simulink model "generatoreqns"  (Simulink 7.6)
settings: Solver=ode45  StartTime=0.0  StopTime=50  RelTol=1e-3
settings Model: Creator=Renata  LastModifiedBy=Renata

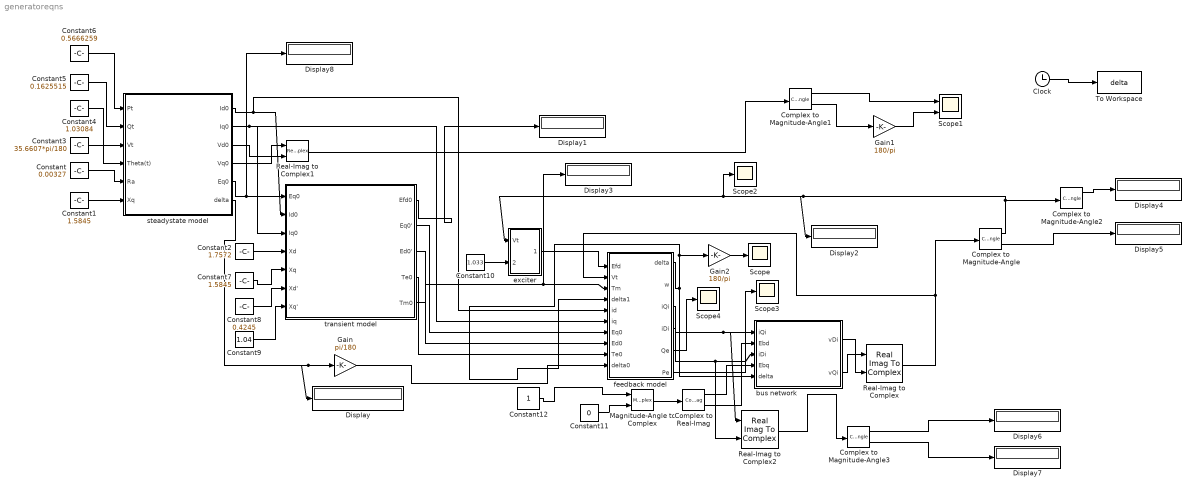
== system generatoreqns ==
  Clock : Clock
      settings: Decimation=10
  Complex to Magnitude-Angle{,1..3} (4 alike) : ComplexToMagnitudeAngle
  Complex to Real-Imag : ComplexToRealImag
  Constant : Constant  Value=0.00327
  Constant1 : Constant  Value=1.5845
  Constant10 : Constant  Value=1.033
  Constant11 : Constant  Value=0
  Constant12 : Constant
  Constant2 : Constant  Value=1.7572
  Constant3 : Constant  Value=35.6607*pi/180
  Constant4 : Constant  Value=1.03084
  Constant5 : Constant  Value=0.1625515
  Constant6 : Constant  Value=0.5666259
  Constant7 : Constant  Value=1.5845
  Constant8 : Constant  Value=0.4245
  Constant9 : Constant  Value=1.04
  Display{,1..8} (9 alike) : Display
  Gain : Gain  Gain=pi/180
  Gain1 : Gain  Gain=180/pi
  Gain2 : Gain  Gain=180/pi
  Magnitude-Angle to Complex : MagnitudeAngleToComplex
  Real-Imag to Complex : RealImagToComplex
  Real-Imag to Complex1 : RealImagToComplex
  Real-Imag to Complex2 : RealImagToComplex
  Scope{,2..4} (4 alike) : Scope
      Scope settings: TickLabels=on  TimeRange=50  YMin=0.85  YMax=1.35
      Scope2 settings: TickLabels=on  TimeRange=50  YMin=0.85  YMax=1.35  SaveName=ScopeData2
      Scope3 settings: TickLabels=on  TimeRange=50  YMin=0.85  YMax=1.35  SaveName=ScopeData3
      Scope4 settings: TickLabels=on  TimeRange=50  YMin=0.85  YMax=1.35  SaveName=ScopeData5
  Scope1 : Scope  NumInputPorts=2
      settings: YMin=-5~-5  YMax=5~5
  To Workspace : ToWorkspace  VariableName=delta  SampleTime=-1  SaveFormat=Structure
      settings: Decimation=100
  bus network : Subsystem
  exciter : Subsystem
  feedback model : Subsystem
  steadystate model : Subsystem
  transient model : Subsystem
  wires:
  steadystate model/1(Id0) -> transient model/2(Id0), feedback model/5(id)
  steadystate model/2(Iq0) -> transient model/3(Iq0), feedback model/6(iq)
  steadystate model/5(Eq0) -> transient model/1(Eq0), Display8/1
  Constant/1 -> steadystate model/5(Ra)
  Constant1/1 -> steadystate model/6(Xq)
  Constant3/1 -> steadystate model/4(Theta(t))
  Constant4/1 -> steadystate model/3(Vt)
  Constant5/1 -> steadystate model/2(Qt)
  Constant6/1 -> steadystate model/1(Pt)
  Constant2/1 -> transient model/4(Xd)
  Constant7/1 -> transient model/5(Xq)
  Constant8/1 -> transient model/6(Xd')
  Constant9/1 -> transient model/7(Xq')
  feedback model/1(delta) -> bus network/5(delta), feedback model/4(delta1), Gain2/1
  Constant10/1 -> exciter/2(Vref)
  feedback model/4(iDi) -> bus network/3(iDi), Real-Imag to Complex2/2
  bus network/1(vDi) -> Real-Imag to Complex/2
  bus network/2(vQi) -> Real-Imag to Complex/1
  Magnitude-Angle to Complex/1 -> Complex to Real-Imag/1
  Constant12/1 -> Magnitude-Angle to Complex/1
  Constant11/1 -> Magnitude-Angle to Complex/2
  Complex to Magnitude-Angle/1 -> Complex to Magnitude-Angle2/1, Display2/1, exciter/1(Vt), Scope2/1
  transient model/1(Efd0) -> Display1/1
  steadystate model/4(Vq0) -> Real-Imag to Complex1/1
  steadystate model/3(Vd0) -> Real-Imag to Complex1/2
  transient model/2(Eq0') -> feedback model/7(Eq0)
  transient model/3(Ed0') -> feedback model/8(Ed0)
  transient model/4(Te0) -> feedback model/9(Te0)
  Real-Imag to Complex1/1 -> Complex to Magnitude-Angle1/1
  steadystate model/6(delta) -> Gain/1, Display/1
  Gain/1 -> feedback model/10(delta0)
  Complex to Magnitude-Angle1/1 -> Scope1/1
  Complex to Magnitude-Angle1/2 -> Gain1/1
  Gain1/1 -> Scope1/2
  feedback model/3(iQi) -> bus network/1(iQi), Real-Imag to Complex2/1
  Real-Imag to Complex/1 -> Complex to Magnitude-Angle/1, feedback model/2(Vt)
  transient model/5(Tm0) -> feedback model/3(Tm), Display3/1
  Complex to Real-Imag/2 -> bus network/2(Ebd)
  Complex to Real-Imag/1 -> bus network/4(Ebq)
  Complex to Magnitude-Angle2/1 -> Display4/1
  Complex to Magnitude-Angle/2 -> Display5/1
  Real-Imag to Complex2/1 -> Complex to Magnitude-Angle3/1
  Complex to Magnitude-Angle3/2 -> Display7/1
  Complex to Magnitude-Angle3/1 -> Display6/1
  Clock/1 -> To Workspace/1
  feedback model/6(Pe) -> Scope3/1
  feedback model/5(Qe) -> Scope4/1
  Gain2/1 -> Scope/1
  exciter/1(Efd) -> feedback model/1(Efd)

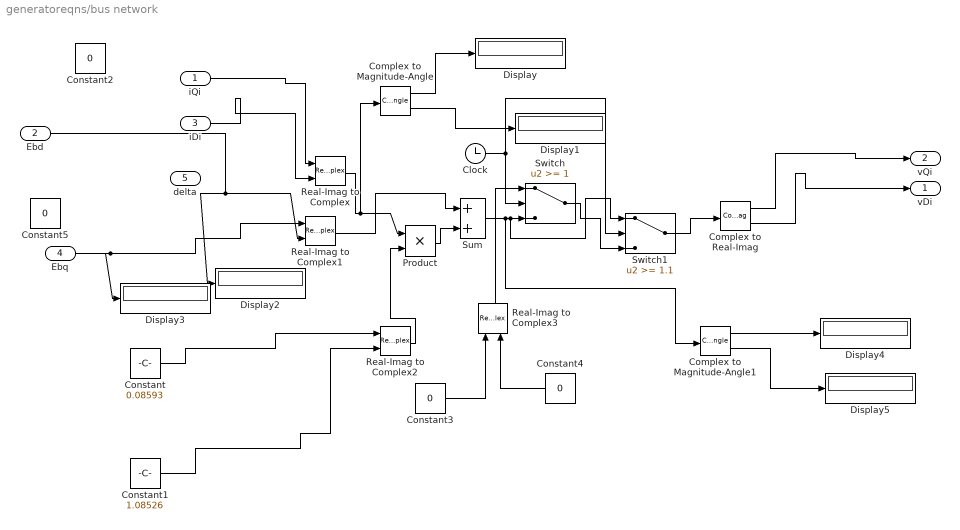
== system generatoreqns/bus network ==
  iQi : Inport
  Ebd : Inport  Port=2
  iDi : Inport  Port=3
  Ebq : Inport  Port=4
  delta : Inport  Port=5
  Clock : Clock
      settings: Decimation=1000
  Complex to Magnitude-Angle : ComplexToMagnitudeAngle
  Complex to Magnitude-Angle1 : ComplexToMagnitudeAngle
  Complex to Real-Imag : ComplexToRealImag
  Constant : Constant  Value=0.08593
  Constant1 : Constant  Value=1.08526
  Constant{2..5} (4 alike) : Constant  Value=0
  Display{,1..5} (6 alike) : Display
  Product : Product  RndMeth=Zero
  Real-Imag to Complex{,1..3} (4 alike) : RealImagToComplex
  Sum : Sum  Inputs=|++
  Switch : Switch  Threshold=1
  Switch1 : Switch  Threshold=1.1
  vDi : Outport
  vQi : Outport  Port=2
  wires:
  Real-Imag to Complex/1 -> Product/1, Complex to Magnitude-Angle/1
  Real-Imag to Complex2/1 -> Product/2
  Product/1 -> Sum/2
  Real-Imag to Complex1/1 -> Sum/1
  Constant/1 -> Real-Imag to Complex2/1
  Constant1/1 -> Real-Imag to Complex2/2
  Switch/1 -> Switch1/3
  iQi/1 -> Real-Imag to Complex/1
  iDi/1 -> Real-Imag to Complex/2
  Clock/1 -> Switch/2, Switch1/2
  Sum/1 -> Complex to Magnitude-Angle1/1, Switch/3, Switch1/1
  Real-Imag to Complex3/1 -> Switch/1
  Constant4/1 -> Real-Imag to Complex3/2
  Constant3/1 -> Real-Imag to Complex3/1
  Complex to Real-Imag/1 -> vQi/1
  Complex to Real-Imag/2 -> vDi/1
  Ebq/1 -> Real-Imag to Complex1/1, Display3/1
  Ebd/1 -> Real-Imag to Complex1/2, Display2/1
  Complex to Magnitude-Angle/1 -> Display/1
  Complex to Magnitude-Angle/2 -> Display1/1
  Complex to Magnitude-Angle1/1 -> Display4/1
  Complex to Magnitude-Angle1/2 -> Display5/1
  Switch1/1 -> Complex to Real-Imag/1

== system generatoreqns/exciter ==
  Vt : Inport
  Vref : Inport  Port=2
  Saturation1 : Saturate  UpperLimit=1.5  LowerLimit=-1.5
  Sum : Sum  Inputs=|+-
  Transfer Fcn : TransferFcn  Numerator=[400]  Denominator=[0.025 1]
  Efd : Outport
  wires:
  Transfer Fcn/1 -> Saturation1/1
  Sum/1 -> Transfer Fcn/1
  Vt/1 -> Sum/1
  Vref/1 -> Sum/2
  Saturation1/1 -> Efd/1

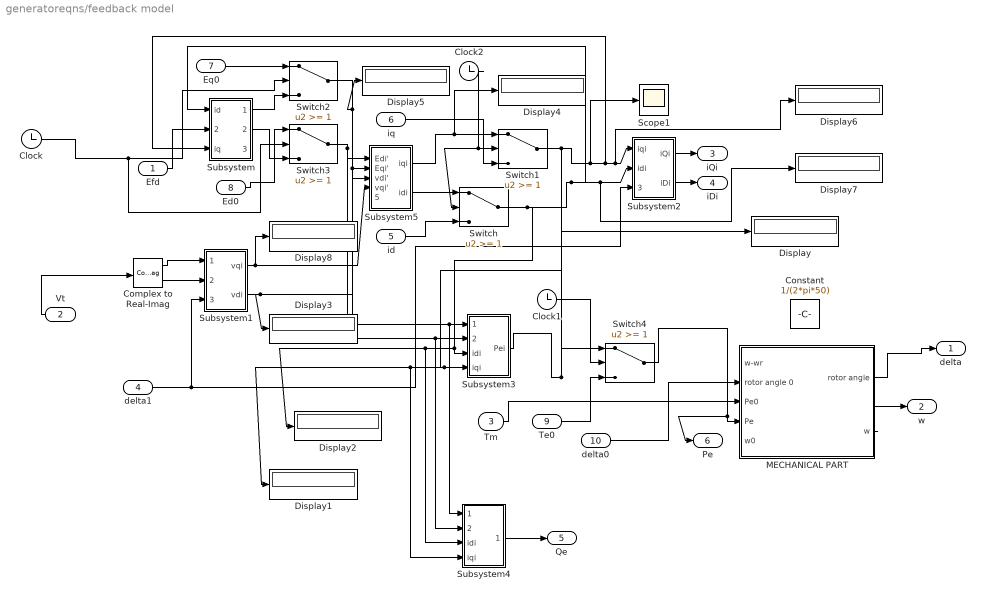
== system generatoreqns/feedback model ==
  Efd : Inport
  Vt : Inport  Port=2
  Tm : Inport  Port=3
  delta1 : Inport  Port=4
  id : Inport  Port=5
  iq : Inport  Port=6
  Eq0 : Inport  Port=7
  Ed0 : Inport  Port=8
  Te0 : Inport  Port=9
  delta0 : Inport  Port=10
  Clock : Clock
      settings: Decimation=1000
  Clock1 : Clock
      settings: Decimation=1000
  Clock2 : Clock
      settings: Decimation=1000
  Complex to Real-Imag : ComplexToRealImag
  Constant : Constant  Value=1/(2*pi*50)
  Display{,1..8} (9 alike) : Display
  MECHANICAL PART : Subsystem
  Scope1 : Scope
      settings: SaveName=ScopeData4
  Subsystem : Subsystem
  Subsystem1 : Subsystem
  Subsystem2 : Subsystem
  Subsystem3 : Subsystem
  Subsystem4 : Subsystem
  Subsystem5 : Subsystem
  Switch{,1..3} (4 alike) : Switch  Threshold=1
  Switch4 : Switch  Threshold=1  ZeroCross=off
  delta : Outport
  w : Outport  Port=2
  iQi : Outport  Port=3
  iDi : Outport  Port=4
  Qe : Outport  Port=5
  Pe : Outport  Port=6
  wires:
  Complex to Real-Imag/1 -> Subsystem1/1(VQi)
  Complex to Real-Imag/2 -> Subsystem1/2(VDi)
  Efd/1 -> Subsystem/2(Efd)
  Vt/1 -> Complex to Real-Imag/1
  Tm/1 -> MECHANICAL PART/3(Pe0)
  Subsystem2/1(iQi) -> iQi/1
  Subsystem2/2(iDi) -> iDi/1
  iq/1 -> Switch1/3
  Clock/1 -> Switch2/2, Switch3/2
  MECHANICAL PART/1(rotor angle) -> delta/1
  MECHANICAL PART/2(w) -> w/1
  delta0/1 -> MECHANICAL PART/2(rotor angle 0)
  Eq0/1 -> Switch2/1
  Subsystem/1(Eqi') -> Switch2/3
  Ed0/1 -> Switch3/1
  Subsystem/2(Edi') -> Switch3/3
  Subsystem5/2(idi) -> Switch/1
  id/1 -> Switch/3
  Subsystem5/1(iqi) -> Switch1/1, Display4/1
  Subsystem3/1(Pei) -> Display/1, Switch4/1
  Switch3/1 -> Subsystem5/1(Edi'), Subsystem3/1(Edi'), Subsystem4/1(Edi')
  Switch2/1 -> Subsystem5/2(Eqi'), Subsystem3/2(Eqi'), Subsystem4/2(Eqi'), Display5/1
  Subsystem1/1(vqi) -> Subsystem5/4(vqi'), Display8/1
  Subsystem1/2(vdi) -> Subsystem5/3(vdi'), Display3/1
  Switch/1 -> Subsystem/1(id), Subsystem2/2(idi), Display7/1, Subsystem3/3(idi), Display2/1, Subsystem4/3(idi)
  Switch1/1 -> Subsystem3/4(iqi), Display1/1, Subsystem4/4(iqi), Subsystem/3(iq), Subsystem2/1(iqi), Display6/1, Scope1/1
  Clock2/1 -> Switch1/2, Switch/2
  delta1/1 -> Subsystem1/3(delta), Subsystem2/3(delta)
  Subsystem4/1(Qei) -> Qe/1
  Te0/1 -> Switch4/3
  Clock1/1 -> Switch4/2
  Switch4/1 -> MECHANICAL PART/4(Pe), Pe/1

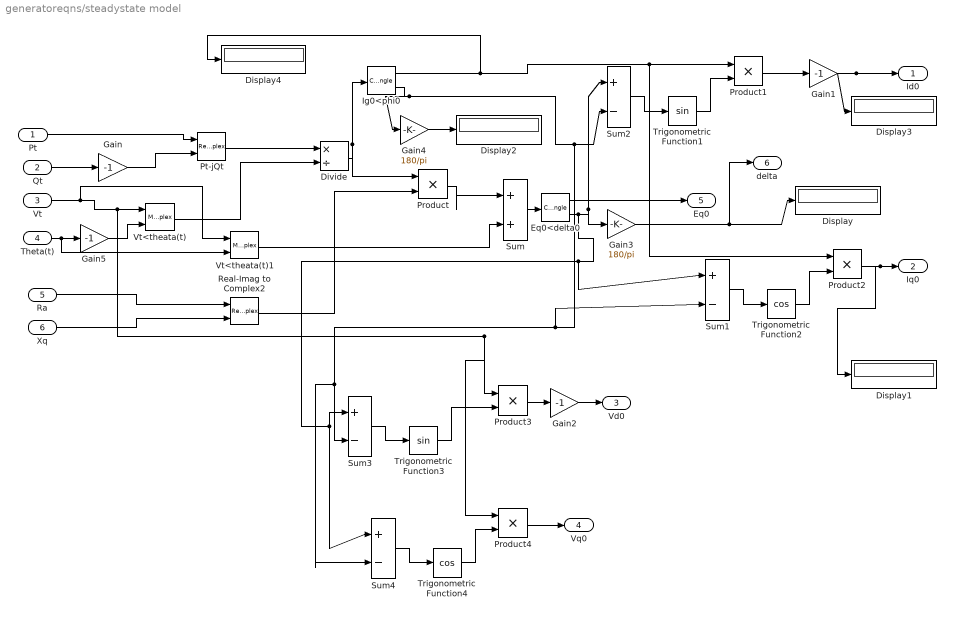
== system generatoreqns/steadystate model ==
  Pt : Inport
  Qt : Inport  Port=2
  Vt : Inport  Port=3
  Theta(t) : Inport  Port=4
  Ra : Inport  Port=5
  Xq : Inport  Port=6
  Display{,1..4} (5 alike) : Display
  Divide : Product  Inputs=*/  RndMeth=Round
  Eq0<delta0 : ComplexToMagnitudeAngle
  Gain{,1..2,5} (4 alike) : Gain  Gain=-1
  Gain3 : Gain  Gain=180/pi
  Gain4 : Gain  Gain=180/pi
  Ig0<phi0 : ComplexToMagnitudeAngle
  Product{,1..4} (5 alike) : Product  RndMeth=Zero
  Pt-jQt : RealImagToComplex
  Real-Imag to Complex2 : RealImagToComplex
  Sum : Sum  Inputs=|++
  Sum{1..4} (4 alike) : Sum  Inputs=|+-
  Trigonometric Function1 : Trigonometry
  Trigonometric Function2 : Trigonometry  Operator=cos
  Trigonometric Function3 : Trigonometry
  Trigonometric Function4 : Trigonometry  Operator=cos
  Vt<theata(t) : MagnitudeAngleToComplex
  Vt<theata(t)1 : MagnitudeAngleToComplex
  Id0 : Outport
  Iq0 : Outport  Port=2
  Vd0 : Outport  Port=3
  Vq0 : Outport  Port=4
  Eq0 : Outport  Port=5
  delta : Outport  Port=6
  wires:
  Qt/1 -> Gain/1
  Gain/1 -> Pt-jQt/2
  Pt/1 -> Pt-jQt/1
  Vt/1 -> Vt<theata(t)/1, Product3/1, Product4/1, Vt<theata(t)1/1
  Pt-jQt/1 -> Divide/1
  Vt<theata(t)/1 -> Divide/2
  Ra/1 -> Real-Imag to Complex2/1
  Xq/1 -> Real-Imag to Complex2/2
  Divide/1 -> Ig0<phi0/1, Product/1
  Real-Imag to Complex2/1 -> Product/2
  Product/1 -> Sum/1
  Sum/1 -> Eq0<delta0/1
  Eq0<delta0/2 -> Sum3/1, Sum4/1, Sum1/1, Sum2/1, Gain3/1
  Sum2/1 -> Trigonometric Function1/1
  Trigonometric Function1/1 -> Product1/2
  Ig0<phi0/1 -> Product1/1, Product2/1, Display4/1
  Product1/1 -> Gain1/1
  Gain1/1 -> Id0/1, Display3/1
  Sum1/1 -> Trigonometric Function2/1
  Trigonometric Function2/1 -> Product2/2
  Product2/1 -> Iq0/1, Display1/1
  Sum3/1 -> Trigonometric Function3/1
  Trigonometric Function3/1 -> Product3/2
  Product3/1 -> Gain2/1
  Gain2/1 -> Vd0/1
  Sum4/1 -> Trigonometric Function4/1
  Trigonometric Function4/1 -> Product4/2
  Product4/1 -> Vq0/1
  Eq0<delta0/1 -> Eq0/1
  Gain3/1 -> Display/1, delta/1
  Ig0<phi0/2 -> Sum2/2, Sum3/2, Sum4/2, Sum1/2, Gain4/1
  Theta(t)/1 -> Gain5/1, Vt<theata(t)1/2
  Gain5/1 -> Vt<theata(t)/2
  Vt<theata(t)1/1 -> Sum/2
  Gain4/1 -> Display2/1

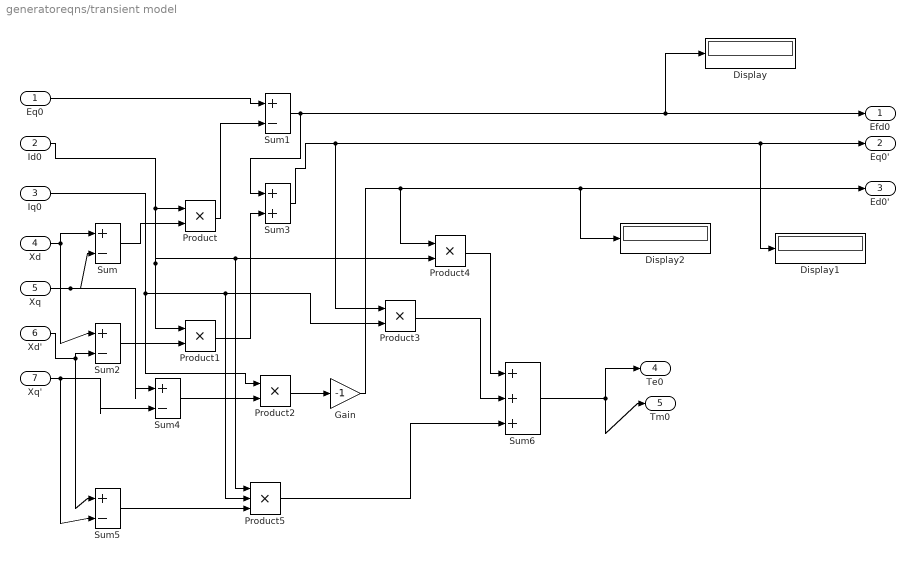
== system generatoreqns/transient model ==
  Eq0 : Inport
  Id0 : Inport  Port=2
  Iq0 : Inport  Port=3
  Xd : Inport  Port=4
  Xq : Inport  Port=5
  Xd' : Inport  Port=6
  Xq' : Inport  Port=7
  Display : Display
  Display1 : Display
  Display2 : Display
  Gain : Gain  Gain=-1
  Product{,1..4} (5 alike) : Product  RndMeth=Zero
  Product5 : Product  Inputs=3  RndMeth=Zero
  Sum{,1..2,4..5} (5 alike) : Sum  Inputs=|+-
  Sum3 : Sum  Inputs=|++
  Sum6 : Sum  Inputs=|+++
  Efd0 : Outport
  Eq0' : Outport  Port=2
  Ed0' : Outport  Port=3
  Te0 : Outport  Port=4
  Tm0 : Outport  Port=5
  wires:
  Sum6/1 -> Te0/1, Tm0/1
  Product5/1 -> Sum6/3
  Product3/1 -> Sum6/2
  Product4/1 -> Sum6/1
  Sum5/1 -> Product5/3
  Gain/1 -> Product4/1, Ed0'/1, Display2/1
  Product2/1 -> Gain/1
  Iq0/1 -> Product2/1, Product3/2, Product5/2
  Sum4/1 -> Product2/2
  Xq'/1 -> Sum4/2, Sum5/2
  Sum3/1 -> Product3/1, Eq0'/1, Display1/1
  Product1/1 -> Sum3/2
  Sum2/1 -> Product1/2
  Xd'/1 -> Sum2/2, Sum5/1
  Sum1/1 -> Sum3/1, Efd0/1, Display/1
  Product/1 -> Sum1/2
  Eq0/1 -> Sum1/1
  Id0/1 -> Product/1, Product1/1, Product4/2, Product5/1
  Sum/1 -> Product/2
  Xq/1 -> Sum/2, Sum4/1
  Xd/1 -> Sum/1, Sum2/1

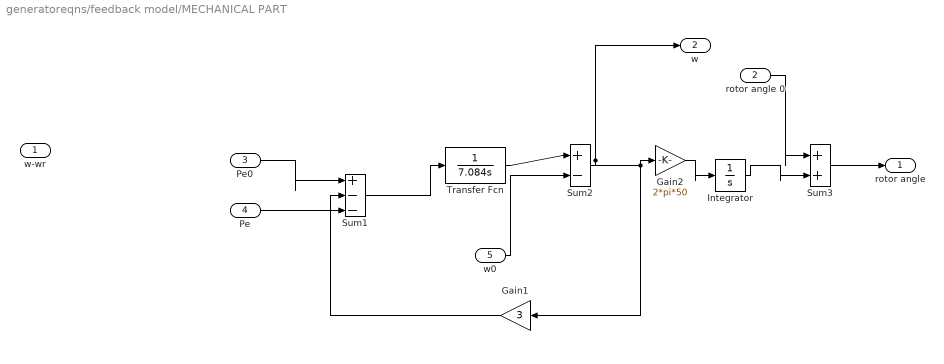
== system generatoreqns/feedback model/MECHANICAL PART ==
  w-wr : Inport
  rotor angle 0 : Inport  Port=2
  Pe0 : Inport  Port=3
  Pe : Inport  Port=4
  w0 : Inport  Port=5
  Gain1 : Gain  Gain=3
  Gain2 : Gain  Gain=2*pi*50
  Integrator : Integrator  ZeroCross=off
  Sum1 : Sum  Inputs=|+--
  Sum2 : Sum  Inputs=|+-
  Sum3 : Sum  Inputs=|++
  Transfer Fcn : TransferFcn  Denominator=[7.084 0]
  rotor angle : Outport
  w : Outport  Port=2
  wires:
  Sum1/1 -> Transfer Fcn/1
  Pe0/1 -> Sum1/1
  Pe/1 -> Sum1/2
  w0/1 -> Sum2/2
  Integrator/1 -> Sum3/2
  Sum3/1 -> rotor angle/1
  Sum2/1 -> w/1, Gain1/1, Gain2/1
  Transfer Fcn/1 -> Sum2/1
  Gain1/1 -> Sum1/3
  Gain2/1 -> Integrator/1
  rotor angle 0/1 -> Sum3/1

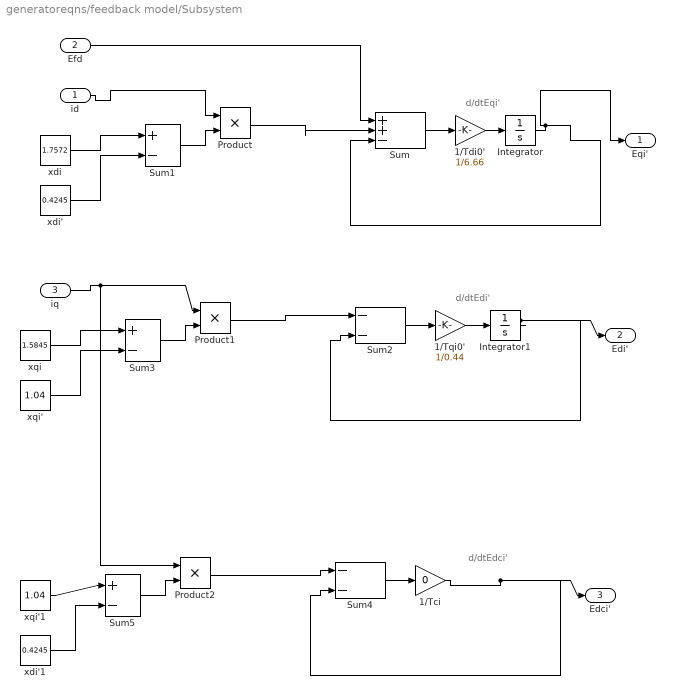
== system generatoreqns/feedback model/Subsystem ==
  note: d/dtEqi'
  note: d/dtEdi'
  note: d/dtEdci'
  id : Inport
  Efd : Inport  Port=2
  iq : Inport  Port=3
  1/Tci : Gain  Gain=0
  1/Tdi0' : Gain  Gain=1/6.66
  1/Tqi0' : Gain  Gain=1/0.44
  Integrator : Integrator
  Integrator1 : Integrator
  Product : Product  RndMeth=Zero
  Product1 : Product  RndMeth=Zero
  Product2 : Product  RndMeth=Zero
  Sum : Sum  Inputs=|++-
  Sum1 : Sum  Inputs=|+-
  Sum2 : Sum  Inputs=--
  Sum3 : Sum  Inputs=|+-
  Sum4 : Sum  Inputs=--
  Sum5 : Sum  Inputs=|+-
  xdi : Constant  Value=1.7572
  xdi' : Constant  Value=0.4245
  xdi'1 : Constant  Value=0.4245
  xqi : Constant  Value=1.5845
  xqi' : Constant  Value=1.04
  xqi'1 : Constant  Value=1.04
  Eqi' : Outport
  Edi' : Outport  Port=2
  Edci' : Outport  Port=3
  wires:
  Integrator/1 -> Eqi'/1, Sum/3
  xdi/1 -> Sum1/1
  xdi'/1 -> Sum1/2
  Sum1/1 -> Product/2
  id/1 -> Product/1
  Product/1 -> Sum/2
  Efd/1 -> Sum/1
  Sum/1 -> 1/Tdi0'/1
  1/Tdi0'/1 -> Integrator/1
  Integrator1/1 -> Edi'/1, Sum2/2
  xqi/1 -> Sum3/1
  xqi'/1 -> Sum3/2
  Sum3/1 -> Product1/2
  iq/1 -> Product1/1, Product2/1
  Sum2/1 -> 1/Tqi0'/1
  1/Tqi0'/1 -> Integrator1/1
  Product1/1 -> Sum2/1
  Sum5/1 -> Product2/2
  Sum4/1 -> 1/Tci/1
  1/Tci/1 -> Edci'/1, Sum4/2
  Product2/1 -> Sum4/1
  xqi'1/1 -> Sum5/1
  xdi'1/1 -> Sum5/2

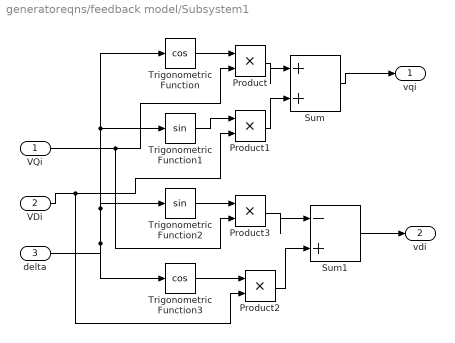
== system generatoreqns/feedback model/Subsystem1 ==
  VQi : Inport
  VDi : Inport  Port=2
  delta : Inport  Port=3
  Product{,1..3} (4 alike) : Product  RndMeth=Zero
  Sum : Sum  Inputs=|++
  Sum1 : Sum  Inputs=|-+
  Trigonometric Function : Trigonometry  Operator=cos
  Trigonometric Function1 : Trigonometry
  Trigonometric Function2 : Trigonometry
  Trigonometric Function3 : Trigonometry  Operator=cos
  vqi : Outport
  vdi : Outport  Port=2
  wires:
  Sum/1 -> vqi/1
  Sum1/1 -> vdi/1
  delta/1 -> Trigonometric Function/1, Trigonometric Function1/1, Trigonometric Function2/1, Trigonometric Function3/1
  Trigonometric Function/1 -> Product/1
  VQi/1 -> Product/2, Product3/2
  Product/1 -> Sum/1
  Trigonometric Function1/1 -> Product1/1
  VDi/1 -> Product1/2, Product2/2
  Product1/1 -> Sum/2
  Trigonometric Function2/1 -> Product3/1
  Trigonometric Function3/1 -> Product2/1
  Product3/1 -> Sum1/1
  Product2/1 -> Sum1/2

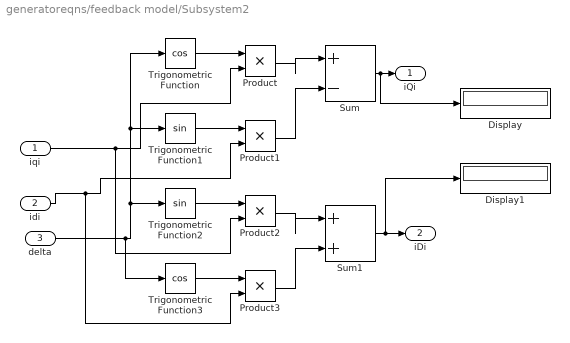
== system generatoreqns/feedback model/Subsystem2 ==
  iqi : Inport
  idi : Inport  Port=2
  delta : Inport  Port=3
  Display : Display
  Display1 : Display
  Product{,1..3} (4 alike) : Product  RndMeth=Zero
  Sum : Sum  Inputs=|+-
  Sum1 : Sum  Inputs=|++
  Trigonometric Function : Trigonometry  Operator=cos
  Trigonometric Function1 : Trigonometry
  Trigonometric Function2 : Trigonometry
  Trigonometric Function3 : Trigonometry  Operator=cos
  iQi : Outport
  iDi : Outport  Port=2
  wires:
  Sum1/1 -> iDi/1, Display1/1
  Sum/1 -> iQi/1, Display/1
  delta/1 -> Trigonometric Function/1, Trigonometric Function1/1, Trigonometric Function2/1, Trigonometric Function3/1
  Trigonometric Function/1 -> Product/1
  iqi/1 -> Product/2, Product2/2
  Product/1 -> Sum/1
  Trigonometric Function1/1 -> Product1/1
  idi/1 -> Product1/2, Product3/2
  Product1/1 -> Sum/2
  Trigonometric Function2/1 -> Product2/1
  Product2/1 -> Sum1/1
  Trigonometric Function3/1 -> Product3/1
  Product3/1 -> Sum1/2

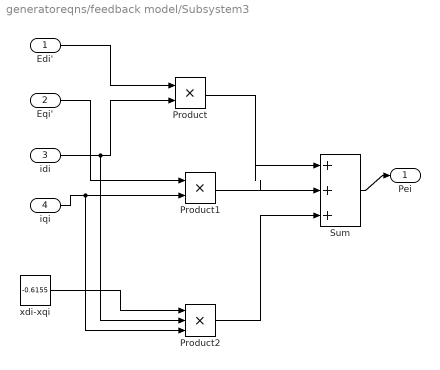
== system generatoreqns/feedback model/Subsystem3 ==
  Edi' : Inport
  Eqi' : Inport  Port=2
  idi : Inport  Port=3
  iqi : Inport  Port=4
  Product : Product  RndMeth=Zero
  Product1 : Product  RndMeth=Zero
  Product2 : Product  Inputs=3  RndMeth=Zero
  Sum : Sum  Inputs=|+++
  xdi-xqi : Constant  Value=-0.6155
  Pei : Outport
  wires:
  idi/1 -> Product/2, Product2/2
  Edi'/1 -> Product/1
  Eqi'/1 -> Product1/1
  iqi/1 -> Product1/2, Product2/3
  xdi-xqi/1 -> Product2/1
  Product/1 -> Sum/1
  Product1/1 -> Sum/2
  Product2/1 -> Sum/3
  Sum/1 -> Pei/1

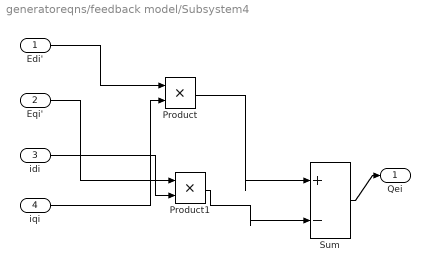
== system generatoreqns/feedback model/Subsystem4 ==
  Edi' : Inport
  Eqi' : Inport  Port=2
  idi : Inport  Port=3
  iqi : Inport  Port=4
  Product : Product  RndMeth=Zero
  Product1 : Product  RndMeth=Zero
  Sum : Sum  Inputs=|+-
  Qei : Outport
  wires:
  Sum/1 -> Qei/1
  Product1/1 -> Sum/2
  Product/1 -> Sum/1
  Eqi'/1 -> Product1/1
  Edi'/1 -> Product/1
  iqi/1 -> Product/2
  idi/1 -> Product1/2

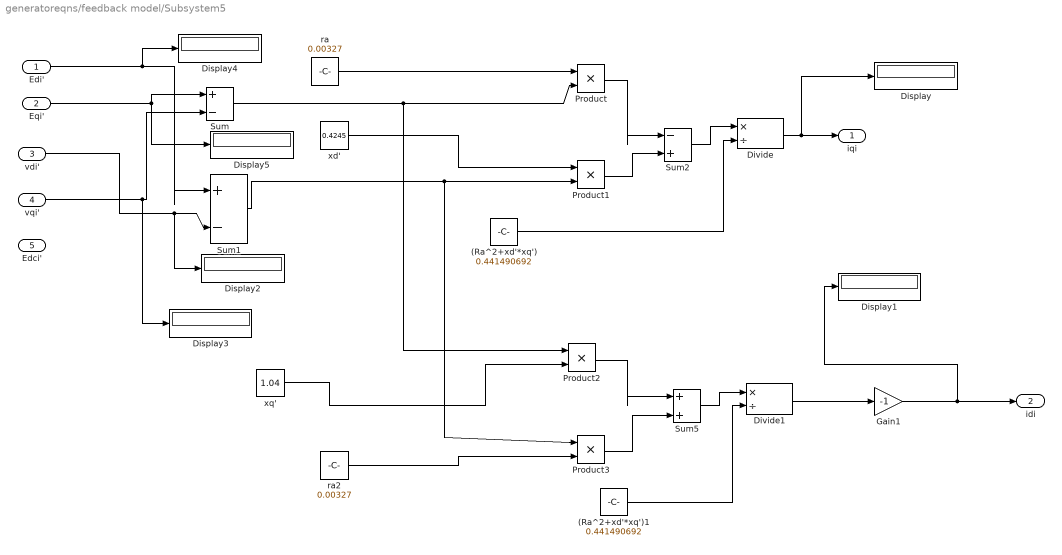
== system generatoreqns/feedback model/Subsystem5 ==
  Edi' : Inport
  Eqi' : Inport  Port=2
  vdi' : Inport  Port=3
  vqi' : Inport  Port=4
  Edci' : Inport  Port=5
  (Ra^2+xd'*xq') : Constant  Value=0.441490692
  (Ra^2+xd'*xq')1 : Constant  Value=0.441490692
  Display{,1..5} (6 alike) : Display
  Divide : Product  Inputs=*/
  Divide1 : Product  Inputs=*/
  Gain1 : Gain  Gain=-1
  Product{,1..3} (4 alike) : Product  RndMeth=Zero
  Sum : Sum  Inputs=|+-
  Sum1 : Sum  Inputs=|+-
  Sum2 : Sum  Inputs=|-+
  Sum5 : Sum  Inputs=|++
  ra : Constant  Value=0.00327
  ra2 : Constant  Value=0.00327
  xd' : Constant  Value=0.4245
  xq' : Constant  Value=1.04
  iqi : Outport
  idi : Outport  Port=2
  wires:
  Eqi'/1 -> Sum/1, Display5/1
  vqi'/1 -> Sum/2, Display3/1
  Sum/1 -> Product/2, Product2/1
  Edi'/1 -> Sum1/1, Display4/1
  vdi'/1 -> Display2/1, Sum1/2
  Sum1/1 -> Product1/2, Product3/1
  Product/1 -> Sum2/1
  Product1/1 -> Sum2/2
  Product2/1 -> Sum5/1
  Product3/1 -> Sum5/2
  ra/1 -> Product/1
  xd'/1 -> Product1/1
  Divide/1 -> iqi/1, Display/1
  (Ra^2+xd'*xq')/1 -> Divide/2
  Sum2/1 -> Divide/1
  xq'/1 -> Product2/2
  ra2/1 -> Product3/2
  Sum5/1 -> Divide1/1
  Divide1/1 -> Gain1/1
  (Ra^2+xd'*xq')1/1 -> Divide1/2
  Gain1/1 -> idi/1, Display1/1
